simulink library "dspmtrx3"  (Simulink 6.0)
settings: Solver=ode45  SolverMode=SingleTasking  StartTime=0.0  StopTime=10.0  RelTol=1e-3
values from neighbouring files (symbols this model uses):
  a = []    [dspfdes.m]    (also in dsprprim.m = a-Mi)
undefined symbols (not defined in the file or in its folder): dTypeID
libraries: dspmtrx3 x12, simulink x3, dspsolvers x3, dspsigattribs x2, dspstat3 x1
settings Model: RequirementInfo=9  CovMetricSettings=d  Creator=szlotkin  LastModifiedBy=mlongfri  ExtModeAutoUpdateStatusClock=off  ProdHWDeviceType=Specified
settings DataIOCC: SignalLoggingName=logsOut
settings OptimizationCC: BooleanDataType=off
settings DebuggingCC: CheckExecutionContextPreStartOutputMsg=on  CheckExecutionContextRuntimeOutputMsg=on  SolverPrmCheckMsg=none
settings HardwareCC: ProdHWDeviceType=Specified  TargetUnknown=on
settings SFSimCC: SFSimApplyToAllLibs=on  SFSimBuildMode=Incremental

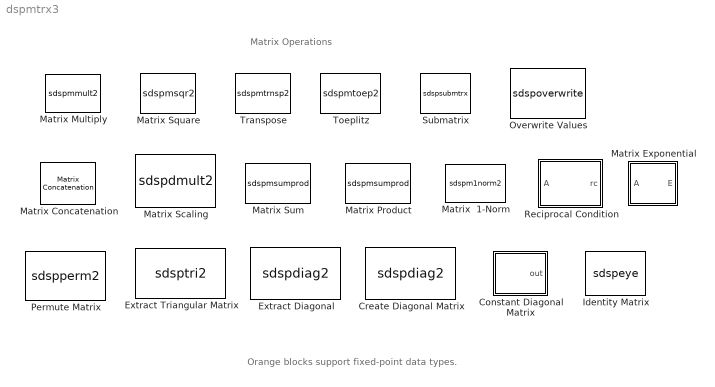
== system dspmtrx3 ==
  note: Matrix Operations
  note: Orange blocks support fixed-point data types.
  Constant Diagonal Matrix : Subsystem  PropExecContextAcrossSSBoundary=on  mask(Constant Diagonal Matrix){q=ones(1,3), frame=off, additionalParams=off, allowOverrides=on, dataType=Inherit from 'Constant(s) along diagonal', isSigned=on, wordLen=16, udDataType=sfix(16), fracBitsMode=Best precision, numFracBits=15}
      mask prompts: q "Constant(s) along diagonal:"; frame "Frame-based output"; additionalParams "------- Show additional parameters --------"; allowOverrides "Allow overrides by DSP Fixed-Point Attributes blocks"; dataType "Output data type:"; isSigned "Signed"; wordLen "Word length:"; udDataType "User-defined data type:"; fracBitsMode "Set fraction length in output to:"; numFracBits "Fraction length:"
      mask help: Generate a diagonal matrix having elements specified by a vector constant.
      mask init:
      | [a,x,y] = dspblkconstdiag('icon',q);
      | dspblkconstdiag('init');
      settings: CopyFcn=dspfixptcopycallback
      mask Help: web(dspbhelp);
      mask StyleString: edit,checkbox,checkbox,checkbox,popup(double|single|int8|uint8|int16|uint16|int32|uint32|boolean|Fixed-point|User-defined|Inherit from 'Constant(s) along diagonal'|Inherit via back propagation),checkbox,edit,edit,popup(Best precision|User-defined),edit
      mask CallbackString: ||||dspblkconstdiag;|||dspblkconstdiag;|dspblkconstdiag;|
      mask TabNameString: Main,Main,Main,Main,Data Types,Data Types,Data Types,Data Types,Data Types,Data Types
      mask Display: plot(x,y)
  Create Diagonal Matrix : S-Function  FunctionName=sdspdiag2  Parameters=mode  mask(Create Diagonal Matrix){}
      mask help: Convert a vector of diagonal elements to a full matrix.
      mask init:
      | mode = 1;
      | x = [.58 .87 .87 .58 .58 NaN 0.45 0.12 NaN 0.525 0.525 0.475 0.475 0.525 0.525 0.565 0.525 ];
      | y = [ 0.2 0.2 0.8 0.8 0.2 NaN 0.2 0.8 NaN 0.435 0.475 0.475 0.525 0.525 0.565 0.5 0.435 ];
      settings: CopyFcn=dspfixptcopycallback
      mask Help: web(dspbhelp);
      mask Display:
      | plot(x,y);
      | port_label('input',1,'D');
      | port_label('output',1,'A');
  Extract Diagonal : S-Function  FunctionName=sdspdiag2  Parameters=mode  mask(Extract Diagonal){}
      mask help: Extract the main diagonal of a full matrix.
      mask init:
      | mode = 2;
      | x = [.58 .87 NaN 0.12 0.45 0.45 0.12 0.12 NaN 0.525 0.525 0.475 0.475 0.525 0.525 0.565 0.525 ];
      | y = [ 0.8 0.2 NaN 0.2 0.2 0.8 0.8 0.2 NaN 0.435 0.475 0.475 0.525 0.525 0.565 0.5 0.435 ];
      settings: CopyFcn=dspfixptcopycallback
      mask Help: web(dspbhelp);
      mask Display:
      | plot(x,y);
      | port_label('input',1,'A');
      | port_label('output',1,'D');
  Extract Triangular Matrix : S-Function  FunctionName=sdsptri2  Parameters=fcn  mask(Extract Triangular Matrix){fcn=Upper}
      mask prompts: fcn "Extract:"
      mask help: Extract upper or lower triangular part of input matrix.
      mask init:
      | [s,x,y] = dspblktri(fcn);
      settings: CopyFcn=dspfixptcopycallback
      mask Help: web(dspbhelp);
      mask StyleString: popup(Upper|Lower)
      mask Display:
      | plot(x,y);
      | port_label('input',1,'A');
      | port_label('output',1,s);
  Identity Matrix : S-Function  FunctionName=sdspeye  Parameters=Inherit,N,Ts,isCustomFloat,isSigned,dTypeID,wordLength,fracBits,1  mask(Identity Matrix){Inherit=off, N=5, Ts=1, additionalParams=off, allowOverrides=on, dataType=double, isSigned=on, wordLen=16, udDataType=sfix(16), fracBitsMode=Best precision, numFracBits=15}
      mask prompts: Inherit "Inherit output port attributes from input port"; N "Matrix size:"; Ts "Sample time:"; additionalParams "------- Show additional parameters --------"; allowOverrides "Allow overrides by DSP Fixed-Point Attributes blocks"; dataType "Output data type:"; isSigned "Signed"; wordLen "Word length:"; udDataType "User-defined data type (e.g. sfix(16), float('single')):"; fracBitsMode "Set fraction length in output to:"; numFracBits "Fraction length:"
      mask help: Output an identity matrix. If the matrix size entered is a scalar, then the output will be a square (symmetric) identity matrix with the number of rows and columns both equal to the specified value. If the matrix size entered is a two-element vector [M N], then the output will be an asymmetric matrix with the number of rows equal to M, the number of columns equal to N, ones down the diagonal, and zeros elsewhere. This matches the syntax of the MATLAB function eye(N) and eye(M,N), respectively.
      mask init:
      | if Inherit,
      |    str = 'eye( )';
      | else
      |    str = ['eye(' ,num2str(&2),')'];
      | end
      | [dtInfo,dTypeID]=dspblkeye('init');
      | isSigned=dtInfo.DataTypeIsSigned;
      | isCustomFloat=dtInfo.DataTypeIsCustomFloat;
      | wordLength=dtInfo.DataTypeWordLength;
      | fracBits=dtInfo.DataTypeFracOrMantBits;
      settings: CopyFcn=dspfixptcopycallback
      mask Help: web(dspbhelp);
      mask StyleString: checkbox,edit,edit,checkbox,checkbox,popup(double|single|int8|uint8|int16|uint16|int32|uint32|boolean|Fixed-point|User-defined|Inherit via back propagation),checkbox,edit,edit,popup(Best precision|User-defined),edit
      mask CallbackString: dspblkeye|||||dspblkeye|||dspblkeye|dspblkeye|
      mask TabNameString: Main,Main,Main,Main,Main,Data Types,Data Types,Data Types,Data Types,Data Types,Data Types
      mask Display: disp(str)
  Matrix Concatenation : simulink/Math Operations/Matrix Concatenation  numInports=2  catMethod=Horizontal
  Matrix Exponential : Subsystem  PropExecContextAcrossSSBoundary=on
      mask Type: Matrix Exponential
      mask Description: Compute the matrix exponential, using a scaling and squaring algorithm with a Pade approximation.  Matrix must be square.
      mask Help: web(dspbhelp);
      mask Display: disp('expm')
  Matrix Product : S-Function  DialogController=dspDDGCreate  DialogControllerArgs=DataTag0  FunctionName=sdspmsumprod  Parameters=Dim,2,dtInfo.interProdMode,dtInfo.interProdWordLength,dtInfo.interProdFracLength,dtInfo.prodOutputMode,dtInfo.prodOutputWordLength,dtInfo.prodOutputFracLength,dtInfo.accumMode,dtInfo.accumWordLength,dtInfo.accumFracLength,dtInfo.outputMode,dtInfo.outputWordLength,dtInfo.outputFracLength,dtInfo.roundingMode,dtInfo.overflowMode  mask(Matrix Product){Dim=Columns, additionalParams=off, allowOverrides=on, outputMode=Same as product output, outputWordLength=16, outputFracLength=15, accumMode=Inherit via internal rule, accumWordLength=32, accumFracLength=30, prodOutputMode=Inherit via internal rule, prodOutputWordLength=32, prodOutputFracLength=30, interProdMode=Same as input, interProdWordLength=16, interProdFracLength=15, roundingMode=Floor, overflowMode=off, LockScale=off}
      mask prompts: Dim "Multiply along:"; additionalParams "------- Show additional parameters -------"; allowOverrides "Allow overrides from DSP Fixed-Point Attributes blocks"; outputMode "Fixed-point output attributes:"; outputWordLength "Output word length:"; outputFracLength "Output fraction length:"; accumMode "Fixed-point accumulator attributes:"; accumWordLength "Accumulator word length:"; accumFracLength "Accumulator fraction length:"; prodOutputMode "Fixed-point product output attributes:"; prodOutputWordLength "Product output word length:"; prodOutputFracLength "Product output fraction length:"; interProdMode "Fixed-point intermediate product attributes:"; interProdWordLength "Intermediate product word length:"; interProdFracLength "Intermediate product fraction length:"; roundingMode "Round integer calculations toward:"; overflowMode "Saturate on integer overflow"; LockScale "Lock scaling"
      mask help:
      | Product of matrix elements along the row or column dimension. Note that 1-D input signals produce a single scalar output equal to the product of the individual elements.
      |
      | The accumulator attributes are only used with complex fixed-point inputs.
      mask init:
      | if (Dim==1), str='Row\nProduct';
      | else str='Column\nProduct';
      | end
      | 
      | %misc         1 USED
      | %output       2 USED
      | %accum        4 USED
      | %prodOutput   8 USED
      | %memory      16
      | %firstCoeff  32
      | %secondCoeff 64
      | %thirdCoeff 128
      | %interProd  256 USED
      | %1+2+4+8+256 = 271
      | dtInfo = dspGetFixptDataTypeInfo(gcbh,271);
      settings: CopyFcn=dspfixptcopycallback
      mask Help: web(dspbhelp);
      mask StyleString: popup(Rows|Columns),checkbox,checkbox,popup(Same as product output|Same as input|Binary point scaling|Slope and bias scaling|User-defined),edit,edit,popup(Inherit via internal rule|Same as product output|Same as input|Binary point scaling|Slope and bias scaling|User-defined),edit,edit,popup(Inherit via internal rule|Same as input|Binary point scaling|Slope and bias scaling|User-defined),edit,edit,popup(Same as input|Binary point scaling|Slope and bias scaling|User-defined),edit,edit,popup(Floor|Nearest),checkbox,checkbox
      mask Display: disp(str);
  Matrix Scaling : S-Function  DialogController=dspDDGCreate  DialogControllerArgs=DataTag1  FunctionName=sdspdmult2  Parameters=mode,D_Source,D_VectFromMask,dtInfo.firstCoeffMode,dtInfo.firstCoeffWordLength,dtInfo.firstCoeffFracLength,dtInfo.prodOutputMode,dtInfo.prodOutputWordLength,dtInfo.prodOutputFracLength,dtInfo.accumMode,dtInfo.accumWordLength,dtInfo.accumFracLength,dtInfo.outputMode,dtInfo.outputWordLength,dtInfo.outputFracLength,dtInfo.roundingMode,dtInfo.overflowMode  mask(Matrix Scaling){mode=Scale Rows (D*A), D_Source=Input port, D_VectFromMask=[0.5 0.25], additionalParams=off, allowOverrides=on, firstCoeffMode=Same word length as input, firstCoeffWordLength=16, firstCoeffFracLength=15, outputMode=Same as product output, outputWordLength=16, outputFracLength=15, accumMode=Inherit via internal rule, accumWordLength=32, accumFracLength=30, prodOutputMode=Inherit via internal rule, prodOutputWordLength=32, prodOutputFracLength=30, roundingMode=Floor, overflowMode=off, LockScale=off}
      mask prompts: D_Source "Scaling vector (D) source:"; D_VectFromMask "Scaling vector (D):"; additionalParams "------- Show additional parameters -------"; allowOverrides "Allow overrides from DSP Fixed-Point Attributes blocks"; firstCoeffMode "Fixed-point scaling vector attributes:"; firstCoeffWordLength "Scaling vector elements word length:"; firstCoeffFracLength "Scaling vector elements fraction length:"; outputMode "Fixed-point output attributes:"; outputWordLength "Output word length:"; outputFracLength "Output fraction length:"; accumMode "Fixed-point accumulator attributes:"; accumWordLength "Accumulator word length"; accumFracLength "Accumulator fraction length:"; prodOutputMode "Fixed-point product output attributes:"; prodOutputWordLength "Product output word length:"; prodOutputFracLength "Product output fraction length:"; roundingMode "Round integer calculations toward:"; overflowMode "Saturate on integer overflow"; LockScale "Lock scaling"
      mask help:
      | Scale the columns or rows of a matrix A by the elements of a vector D.  This is equivalent to multiplying a full matrix (A) by a diagonal (D), and vice versa. Note that unoriented input signals are treated as oriented column vectors. The output of this block is always oriented.
      |
      | For some fixed-point modes, the scaling vector fraction length or slope is automatically set for you to ''Best precision.'' In these cases, the scaling is set to the best possible precision given the scaling vector real-world values and word length. This is equivalent to the ''Best Precision: Matrix-wise'' scaling option used in some Simulink fixed-point blocks.
      |
      | The accumulator attributes on the ''Fixed-point'' tab are only used with complex fixed-point inputs.
      mask init:
      | %misc         1 USED
      | %output       2 USED
      | %accum        4 USED
      | %prodOutput   8 USED
      | %memory      16
      | %firstCoeff  32 USED
      | %1+2+4+8+256 = 47
      | dtInfo = dspGetFixptDataTypeInfo(gcbh,47);
      | 
      | if (strcmp(mode,'Scale rows (D*A)'))
      |     s = 'Scale\nRows\nD*A';
      | else
      | 	s = 'Scale\nColumns\nA*D';
      | end
      | 
      | inp1_index = 1;
      | inp1_label = 'A';
      | if (D_Source == 1),
      |   inp2_index = 2;
      |   inp2_label = 'D';
      | else
      |   inp2_index = 1;
      |   inp2_label = 'A';
      | end
      settings: CopyFcn=dspfixptcopycallback
      mask Help: web(dspbhelp);
      mask StyleString: popup(Scale rows (D*A)|Scale columns (A*D)),popup(Input port|Dialog parameter),edit,checkbox,checkbox,popup(Same word length as input|Specify word length|Binary point scaling|Slope and bias scaling|User-defined),edit,edit,popup(Same as product output|Same as first input|Binary point scaling|Slope and bias scaling|User-defined),edit,edit,popup(Inherit via internal rule|Same as product output|Same as first input|Binary point scaling|Slope and bias scaling|User-defined),edit,edit,popup(Inherit via internal rule|Same as first input|Binary point scaling|Slope and bias scaling|User-defined),edit,edit,popup(Floor|Nearest),checkbox,checkbox
      mask Display:
      | port_label('input',inp1_index,inp1_label);
      | port_label('input',inp2_index,inp2_label);
      | disp(s);
  Matrix Square : S-Function  FunctionName=sdspmsqr2
      mask Type: Matrix Square
      mask Description: Compute the matrix square, U' * U.  Hermitian transpose is performed for complex inputs.  [Mx1] and [1xN] input matrices may be used to compute efficient outer and inner products, respectively. Vector input signals are treated as [Mx1] matrices. The output is always a matrix.
      mask Help: web(dspbhelp);
      mask Display: disp('u^Hu','texmode','on')
  Matrix Sum : S-Function  DialogController=dspDDGCreate  DialogControllerArgs=DataTag2  FunctionName=sdspmsumprod  Parameters=Dim,1,-1,0,0,-1,0,0,dtInfo.accumMode,dtInfo.accumWordLength,dtInfo.accumFracLength,dtInfo.outputMode,dtInfo.outputWordLength,dtInfo.outputFracLength,dtInfo.roundingMode,dtInfo.overflowMode  mask(Matrix Sum){Dim=Columns, additionalParams=off, allowOverrides=on, outputMode=Same as accumulator, outputWordLength=16, outputFracLength=15, accumMode=Inherit via internal rule, accumWordLength=32, accumFracLength=30, roundingMode=Floor, overflowMode=off, LockScale=off}
      mask prompts: Dim "Sum along:"; additionalParams "------- Show additional parameters -------"; allowOverrides "Allow overrides from DSP Fixed-Point Attributes blocks"; outputMode "Fixed-point output attributes:"; outputWordLength "Output word length:"; outputFracLength "Output fraction length:"; accumMode "Fixed-point accumulator attributes:"; accumWordLength "Accumulator word length:"; accumFracLength "Accumulator fraction length:"; roundingMode "Round integer calculations toward:"; overflowMode "Saturate on integer overflow"; LockScale "Lock scaling"
      mask help: Sum of matrix elements along the row or column dimension. Note that 1-D input signals produce a single scalar output equal to the sum of the individual elements.
      mask init:
      | if (Dim==1), str='Row\nSum';
      | else str='Column\nSum';
      | end
      | 
      | %misc       1 USED
      | %output     2 USED
      | %accum      4 USED
      | dtInfo = dspGetFixptDataTypeInfo(gcbh,7);
      settings: CopyFcn=dspfixptcopycallback
      mask Help: web(dspbhelp);
      mask StyleString: popup(Rows|Columns),checkbox,checkbox,popup(Same as accumulator|Same as input|Binary point scaling|Slope and bias scaling|User-defined),edit,edit,popup(Inherit via internal rule|Same as input|Binary point scaling|Slope and bias scaling|User-defined),edit,edit,popup(Floor|Nearest),checkbox,checkbox
      mask Display: disp(str);
  Matrix  1-Norm : S-Function  DialogController=dspDDGCreate  DialogControllerArgs=DataTag3  FunctionName=sdspm1norm2  Parameters=dtInfo.accumMode,dtInfo.accumWordLength,dtInfo.accumFracLength,dtInfo.outputMode,dtInfo.outputWordLength,dtInfo.outputFracLength,dtInfo.roundingMode,dtInfo.overflowMode  mask(Matrix 1-Norm){allowOverrides=on, outputMode=Same as accumulator, outputWordLength=16, outputFracLength=15, accumMode=Inherit via internal rule, accumWordLength=32, accumFracLength=30, roundingMode=Floor, overflowMode=off, LockScale=off}
      mask prompts: allowOverrides "Allow overrides from DSP Fixed-Point Attributes blocks"; outputMode "Fixed-point output attributes:"; outputWordLength "Output word length:"; outputFracLength "Output fraction length:"; accumMode "Fixed-point accumulator attributes:"; accumWordLength "Accumulator word length:"; accumFracLength "Accumulator fraction length:"; roundingMode "Round integer calculations toward:"; overflowMode "Saturate on integer overflow"; LockScale "Lock scaling"
      mask help: Compute the matrix 1-norm, which is the largest column sum of absolute values. Note that unoriented input signals are treated as oriented column vectors. The output of this block is always oriented.
      mask init:
      | dtInfo = dspGetFixptDataTypeInfo(gcbh,7);
      settings: CopyFcn=dspfixptcopycallback
      mask Help: web(dspbhelp);
      mask StyleString: checkbox,popup(Same as accumulator|Same as input|Binary point scaling|Slope and bias scaling|User-defined),edit,edit,popup(Inherit via internal rule|Same as input|Binary point scaling|Slope and bias scaling|User-defined),edit,edit,popup(Floor|Nearest),checkbox,checkbox
      mask Display: disp('Matrix\n1-Norm')
  Matrix Multiply : S-Function  FunctionName=sdspmmult2  Parameters=numInputPorts,OptimizationLevel  mask(Matrix Multiply){numInputPorts=2, OptimizationLevel=None}
      mask prompts: numInputPorts "Number of input ports:"; OptimizationLevel "Optimization:"
      mask help: Multiply input matrices.
      mask init:
      | dspblkmmult(numInputPorts);
      mask Help: web(dspbhelp);
      mask StyleString: edit,popup(None|Memory|Flops)
      mask Display: port_label('input',1, 'A'); port_label('input',2, 'B'); port_label('output', 1, 'A*B');
  Overwrite Values : S-Function  FunctionName=sdspoverwrite  Parameters=ColSpan, ColStartMode, ColStartIndex, ColEndMode, ColEndIndex, RowSpan, RowStartMode, RowStartIndex, RowEndMode, RowEndIndex, OverWriteDiag, ConstValue, DiagSpan, DiagStartMode, DiagStartIndex, DiagEndMode, DiagEndIndex, valFrom2ndIP  mask(Overwrite Values){OverWriteDiag=Submatrix, valFrom2ndIP=Specify via dialog, ConstValue=0, RowSpan=Range of rows, RowStartMode=First, RowStartIndex=1, RowEndMode=Last, RowEndIndex=1, ColSpan=Range of columns, ColStartMode=First, ColStartIndex=1, ColEndMode=Last, ColEndIndex=1, DiagSpan=Range of elements, DiagStartMode=Index, DiagStartIndex=2, DiagEndMode=Index, DiagEndIndex=4}
      mask prompts: OverWriteDiag "Overwrite:"; valFrom2ndIP "Source of overwriting value(s):"; ConstValue "Overwrite with:"; RowSpan "Row span:"; RowStartMode "Starting row:"; RowStartIndex "Starting row index:"; RowEndMode "Ending row:"; RowEndIndex "Ending row index:"; ColSpan "Column span:"; ColStartMode "Starting column:"; ColStartIndex "Starting column index:"; ColEndMode "Ending column:"; ColEndIndex "Ending column index:"; DiagSpan "Diagonal span:"; DiagStartMode "Starting element:"; DiagStartIndex "Starting element index:"; DiagEndMode "Ending element:"; DiagEndIndex "Ending element index:"
      mask help:
      | Overwrites a selected portion of the input matrix--either a submatrix, full diagonal, or a portion of the diagonal.
      | Specify overwriting values as follows:
      |   --Matrix with the same dimensions as the submatrix
      |   --Vector with the same length as the portion of the diagonal
      |   --Scalar constant with which to replace each element in the submatrix or diagonal portion.
      |
      | Treats unoriented (1-D) input vectors as column vectors.
      mask init:
      | [x1,y1,xc,yc,xmc,ymc,xi,yi] = dspblkoverwrite('icon');
      | if valFrom2ndIP == 1
      |   i1=1;
      |   s1='';
      | else
      |   i1=2;
      |   s1='V';
      | end;
      settings: CopyFcn=dspfixptcopycallback
      mask Help: web(dspbhelp);
      mask StyleString: popup(Submatrix|Diagonal),popup(Specify via dialog|Second input port),edit,popup(All rows|One row|Range of rows),popup(First|Index|Offset from last|Last|Offset from middle|Middle),edit,popup(Index|Offset from last|Last|Offset from middle|Middle),edit,popup(All columns|One column|Range of columns),popup(First|Index|Offset from last|Last|Offset from middle|Middle),edit,popup(Index|Offset from last|Last|Offset from middle|Middle),edit,popup(All elements|One element|Range of elements),popup(First|Index|Offset from last|Last|Offset from middle|Middle),edit,popup(Index|Offset from last|Last|Offset from middle|Middle),edit
      mask CallbackString:
      | dspblkoverwrite;
      | dspblkoverwrite('icon');|dspblkoverwrite||dspblkoverwrite|dspblkoverwrite||dspblkoverwrite||dspblkoverwrite|dspblkoverwrite||dspblkoverwrite||dspblkoverwrite|dspblkoverwrite||dspblkoverwrite|
      mask Display:
      | plot(x1,y1,xc,yc,xmc,ymc,xi,yi);
      | port_label('input',1,'A');
      | port_label('output',1,'B');
      | port_label('input',i1,s1);
  Permute Matrix : S-Function  FunctionName=sdspperm2  Parameters=mode,errmode,checkDims, ZeroOneIdxMode  mask(Permute Matrix){mode=Columns, ZeroOneIdxMode=One-based, errmode=Clip Index, checkDims=off}
      mask prompts: mode "Permute:"; ZeroOneIdxMode "Index mode:"; errmode "Invalid permutation index:"; checkDims "Error when length of P is not equal to Permute dimension size"
      mask help: Permutes the rows or columns of a matrix or vector A, based on a vector P of integer-valued permutation indices. The indices need not be unique. When you select the Error check box, the length of vector P must be the same as the number of input rows or columns (whichever you are permuting).
      settings: CopyFcn=dspfixptcopycallback
      mask Help: web(dspbhelp);
      mask StyleString: popup(Rows|Columns),popup(Zero-based|One-based),popup(Clip Index|Clip and Warn|Generate Error),checkbox
      mask Display:
      | disp(['Permute\n' &1]);
      | port_label('input',1,'A');
      | port_label('input',2,'P');
  Reciprocal Condition : Subsystem  PropExecContextAcrossSSBoundary=on
      mask Type: Reciprocal Condition
      mask Description: Estimates the reciprocal of the condition of a square input matrix in the 1-norm.  If input is well conditioned, the output is near 1.0.  If input is badly conditioned, output is near 0.0.
      mask Help: web(dspbhelp);
      mask Display: disp('RCond')
  Submatrix : S-Function  FunctionName=sdspsubmtrx  Parameters=ColSpan, ColStartMode, ColStartIndex, ColEndMode, ColEndIndex, RowSpan, RowStartMode, RowStartIndex, RowEndMode, RowEndIndex  mask(Submatrix){RowSpan=Range of rows, RowStartMode=First, RowStartIndex=1, RowEndMode=Last, RowEndIndex=1, ColSpan=Range of columns, ColStartMode=First, ColStartIndex=1, ColEndMode=Last, ColEndIndex=1}
      mask prompts: RowSpan "Row span:"; RowStartMode "Starting row:"; RowStartIndex "Starting row index:"; RowEndMode "Ending row:"; RowEndIndex "Ending row index:"; ColSpan "Column span:"; ColStartMode "Starting column:"; ColStartIndex "Starting column index:"; ColEndMode "Ending column:"; ColEndIndex "Ending column index:"
      mask help: Return selected portion of input matrix. 1-D input signals are treated as 2-D column vectors. The output is always 2-D.
      mask init:
      | [x1,y1,xc,yc,xi,yi] = dspblksubmatrix('icon');
      settings: CopyFcn=dspfixptcopycallback
      mask Help: web(dspbhelp);
      mask StyleString: popup(All rows|One row|Range of rows),popup(First|Index|Offset from last|Last|Offset from middle|Middle),edit,popup(Index|Offset from last|Last|Offset from middle|Middle),edit,popup(All columns|One column|Range of columns),popup(First|Index|Offset from last|Last|Offset from middle|Middle),edit,popup(Index|Offset from last|Last|Offset from middle|Middle),edit
      mask CallbackString: dspblksubmatrix|dspblksubmatrix||dspblksubmatrix||dspblksubmatrix|dspblksubmatrix||dspblksubmatrix|
      mask Display: plot(x1,y1,xc,yc,xi,yi);
  Toeplitz : S-Function  FunctionName=sdspmtoep2  Parameters=Symmetric,1,overflowFlag+1  mask(Toeplitz){Symmetric=on, overflowFlag=on}
      mask prompts: overflowFlag "Saturate on integer overflow"
      mask help: Generate a symmetric or asymmetric Toeplitz matrix. If Symmetric is selected, a symmetric (or Hermitian) Toeplitz matrix is generated. If Symmetric is not selected, an asymmetric Toeplitz matrix is generated. The columns and rows are specified by the first and second inputs, respectively. The first matrix element is inherited from the column.
      mask init:
      | if (Symmetric==1)
      |   % Do not display anything on ports for this case
      |   p1 = 1; L1 = '';
      |   p2 = 1;  L2 = '';
      |   % Icon display is diagonal matrix picture
      |   horiz_offset = 0.1;
      |   xm=horiz_offset + .8*[0.25 0.1625 0.1625 0.25 NaN 0.7875 0.8875 0.8875 0.7875 NaN 0.25 0.75 NaN 0.4125 0.75 NaN 0.5875 0.75 NaN 0.25 0.5875 NaN 0.25 0.4125];
      |   ym=[.9 .9 .1 .1 NaN .9 .9 .1 .1 NaN .8 .2 NaN .8 .4 NaN .8 .6 NaN .6 .2 NaN .4 .2];
      | else
      |   p1 = 1;  L1 = 'Toep Col';
      |   p2 = 2;  L2 = 'Toep Row';
      |   % Icon display is blank
      |   xm = 0;
      |   ym = 0;
      | end
      settings: CopyFcn=dspfixptcopycallback
      mask Help: web(dspbhelp);
      mask CallbackString:
      | if (strcmp(get_param(gcbh,'Symmetric'),'on'))
      | 	set_param(gcbh,'MaskVisibilities',{'on','on'})
      | else
      | 	set_param(gcbh,'MaskVisibilities',{'on','off'})
      | end|
      mask Display:
      | plot(xm,ym);
      | port_label('input', p1, L1);
      | port_label('input', p2, L2);
  Transpose : S-Function  FunctionName=sdspmtrnsp2  Parameters=Hermitian,1,overflowFlag+1  mask(Transpose){Hermitian=off, overflowFlag=on}
      mask prompts: overflowFlag "Saturate on integer overflow"
      mask help: Compute the matrix transpose. Vector input signals are treated as [Mx1] matrices. The output is always a matrix.
      mask init:
      | if(Hermitian==1),  str = 'u^H';
      | else               str = 'u^T';
      | end
      settings: CopyFcn=dspfixptcopycallback
      mask Help: web(dspbhelp);
      mask CallbackString:
      | if (strcmp(get_param(gcbh,'Hermitian'),'on'))
      | 	set_param(gcbh,'MaskVisibilities',{'on','on'});
      | else
      | 	set_param(gcbh,'MaskVisibilities',{'on','off'});
      | end|
      mask Display: disp(str,'texmode','on')

== system dspmtrx3/Constant Diagonal Matrix ==
  Constant : Constant  Value=a
  Frame Status Conversion : dspsigattribs/Frame Status Conversion  growRefPort=off  outframe=Sample-based
  out : Outport  InitialOutput=0
  wires:
  Constant/1 -> Frame Status Conversion/1
  Frame Status Conversion/1 -> out/1

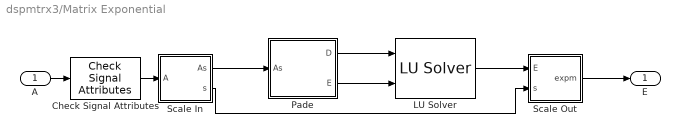
== system dspmtrx3/Matrix Exponential ==
  A : Inport  LatchInput=off
  Check Signal Attributes : dspsigattribs/Check Signal Attributes  SigAttribCheckMethod=Does not match attributes exactly  Complexity=Ignore  Frame=Sample-based  DimsCheckMethod=Is...  Dimensions=Square matrix (2-D)  DatatypeCheckMethod=Is...  DatatypeGeneral=Floating-point  DtypeFloatSpecific=Any floating-point  DtypeFixedSpecific=Any fixed-point  DtypeIntSpecific=Any integer  SampleMode=Ignore
  LU Solver : dspsolvers/LU Solver
  Pade : Subsystem  PropExecContextAcrossSSBoundary=on
      mask Display: disp('Pade\nApprox')
  Scale In : Subsystem  PropExecContextAcrossSSBoundary=on
  Scale Out : Subsystem  PropExecContextAcrossSSBoundary=on
  E : Outport
  wires:
  Check Signal Attributes/1 -> Scale In/1(A)
  A/1 -> Check Signal Attributes/1
  Scale In/1(As) -> Pade/1(As)
  Scale Out/1(expm) -> E/1
  Scale In/2(s) -> Scale Out/2(s)
  Pade/2(E) -> LU Solver/2
  Pade/1(D) -> LU Solver/1
  LU Solver/1 -> Scale Out/1(E)

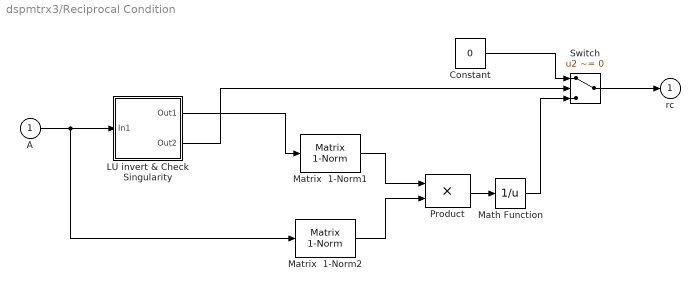
== system dspmtrx3/Reciprocal Condition ==
  A : Inport  LatchInput=off
  Constant : Constant  Value=0
  LU invert & Check Singularity : Subsystem  PropExecContextAcrossSSBoundary=on
      mask Display:
      | port_label('output',1,'Inv');
      | port_label('output',2,'Status');
      | port_label('input',1,'Mx');
  Math Function : Math  Operator=reciprocal  SaturateOnIntegerOverflow=on
  Matrix  1-Norm1 : dspmtrx3/Matrix  1-Norm
  Matrix  1-Norm2 : dspmtrx3/Matrix  1-Norm
  Product : Product  SaturateOnIntegerOverflow=on  InputSameDT=on
  Switch : Switch  Criteria=u2 ~= 0  InputSameDT=on
  " rc" : Outport  InitialOutput=0
  wires:
  LU invert & Check Singularity/2(Out2) -> Switch/2
  Math Function/1 -> Switch/3
  Switch/1 -> " rc"/1
  Product/1 -> Math Function/1
  Matrix  1-Norm2/1 -> Product/2
  Matrix  1-Norm1/1 -> Product/1
  Constant/1 -> Switch/1
  LU invert & Check Singularity/1(Out1) -> Matrix  1-Norm1/1
  A/1 -> LU invert & Check Singularity/1(In1), Matrix  1-Norm2/1

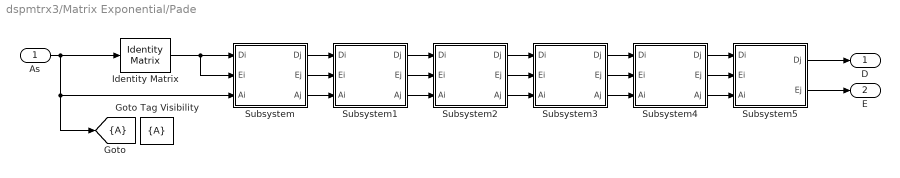
== system dspmtrx3/Matrix Exponential/Pade ==
  As : Inport  LatchInput=off
  Goto Tag Visibility : GotoTagVisibility
  Identity Matrix : dspmtrx3/Identity Matrix  Inherit=on  N=5  Ts=1  dataType=double  wordLen=16  udDataType=sfix(16)  fracBitsMode=Best precision  numFracBits=15
  Subsystem : Subsystem  PropExecContextAcrossSSBoundary=on
      mask Display: disp('Pade\n1')
  Subsystem1 : Subsystem  PropExecContextAcrossSSBoundary=on
      mask Display: disp('Pade\n2')
  Subsystem2 : Subsystem  PropExecContextAcrossSSBoundary=on
      mask Display: disp('Pade\n3')
  Subsystem3 : Subsystem  PropExecContextAcrossSSBoundary=on
      mask Display: disp('Pade\n4')
  Subsystem4 : Subsystem  PropExecContextAcrossSSBoundary=on
      mask Display: disp('Pade\n5')
  Subsystem5 : Subsystem  PropExecContextAcrossSSBoundary=on
      mask Display: disp('Pade\n6')
  D : Outport
  E : Outport  Port=2
  tag scope: A=scoped
  wires:
  As/1 -> Identity Matrix/1, Subsystem/3(Ai), [A]
  Identity Matrix/1 -> Subsystem/1(Di), Subsystem/2(Ei)
  Subsystem/1(Dj) -> Subsystem1/1(Di)
  Subsystem/2(Ej) -> Subsystem1/2(Ei)
  Subsystem1/1(Dj) -> Subsystem2/1(Di)
  Subsystem1/2(Ej) -> Subsystem2/2(Ei)
  Subsystem2/1(Dj) -> Subsystem3/1(Di)
  Subsystem2/2(Ej) -> Subsystem3/2(Ei)
  Subsystem3/1(Dj) -> Subsystem4/1(Di)
  Subsystem3/2(Ej) -> Subsystem4/2(Ei)
  Subsystem4/1(Dj) -> Subsystem5/1(Di)
  Subsystem4/2(Ej) -> Subsystem5/2(Ei)
  Subsystem5/2(Ej) -> E/1
  Subsystem5/1(Dj) -> D/1
  Subsystem/3(Aj) -> Subsystem1/3(Ai)
  Subsystem1/3(Aj) -> Subsystem2/3(Ai)
  Subsystem2/3(Aj) -> Subsystem3/3(Ai)
  Subsystem3/3(Aj) -> Subsystem4/3(Ai)
  Subsystem4/3(Aj) -> Subsystem5/3(Ai)

== system dspmtrx3/Matrix Exponential/Scale In ==
  A : Inport  LatchInput=off
  Inf norm : Subsystem  PropExecContextAcrossSSBoundary=on
      mask Display: disp('inf\nnorm')
  Pow2 Scaling : Subsystem  PropExecContextAcrossSSBoundary=on
      mask Display: disp('s-scaling')
  Scale Input : Subsystem  PropExecContextAcrossSSBoundary=on
  log2 : Subsystem  PropExecContextAcrossSSBoundary=on
      mask Display: disp('log2')
  As : Outport
  s : Outport  Port=2
  wires:
  A/1 -> Inf norm/1(In1), Scale Input/2(A)
  Inf norm/1(Out1) -> log2/1(u)
  log2/1(e) -> Pow2 Scaling/1(In1)
  Pow2 Scaling/1(Out1) -> Scale Input/1(s), s/1
  Scale Input/1(sA) -> As/1

== system dspmtrx3/Matrix Exponential/Scale Out ==
  E : Inport  LatchInput=off
  s : Inport  Port=2  LatchInput=off
  Matrix Squaring : Subsystem  TreatAsAtomicUnit=on  PropExecContextAcrossSSBoundary=on
  Switch : Switch  Criteria=u2 ~= 0  SaturateOnIntegerOverflow=on
  expm : Outport
  wires:
  s/1 -> Matrix Squaring/2(N), Switch/2
  E/1 -> Matrix Squaring/1(E), Switch/3
  Matrix Squaring/1(Out) -> Switch/1
  Switch/1 -> expm/1

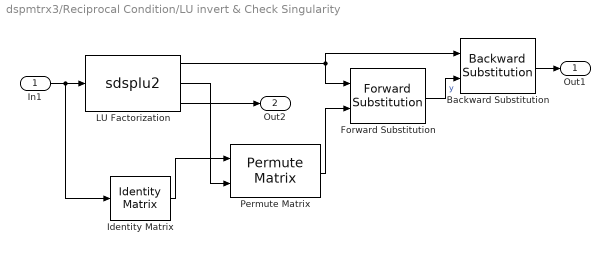
== system dspmtrx3/Reciprocal Condition/LU invert & Check Singularity ==
  In1 : Inport  LatchInput=off
  Backward Substitution : dspsolvers/Backward Substitution  unit=off
  Forward Substitution : dspsolvers/Forward Substitution  unit=on
  Identity Matrix : dspmtrx3/Identity Matrix  Inherit=on  N=5  Ts=1  dataType=double  wordLen=16  udDataType=sfix(16)  fracBitsMode=Best precision  numFracBits=15
  LU Factorization : S-Function  AncestorBlock=dspfactors/LU Factorization  FunctionName=sdsplu2  Parameters=singular  mask(LU Factorization){singular=on}
      mask prompts: singular "Show singularity  status"
      mask help: LU factorization with row pivoting. Only for use with a square input matrix A. Stores L (a unit-lower triangular matrix) in the lower triangle and U in the upper triangle of the output matrix. Permutation vector P is output separately.
      mask init:
      | x=[ 0.58 0.85 0.58 0.58 NaN 0.895 0.625 0.895 0.895 NaN 0.12 0.45 0.45 0.12 0.12 NaN 0.525 0.525 0.475 0.475 0.525 0.525 0.565 0.525 ];
      | y=[ 0.1 0.1 0.7 0.1 NaN 0.1 0.7 0.7 0.1 NaN 0.1 0.1 0.7 0.7 0.1 NaN 0.335 0.375 0.375 0.425 0.425 0.465 0.4 0.335 ];
      mask Help: web(dspbhelp);
      mask Display:
      | plot(x,y); text(.25,0.9,'P A = L U')
      | port_label('input',1,'A');
      | port_label('output',1,'LU');
      | port_label('output',2,'P');
      | port_label('output',3,'S');
  Permute Matrix : dspmtrx3/Permute Matrix  mode=Rows  ZeroOneIdxMode=One-based  errmode=Clip Index  checkDims=on
  Out1 : Outport
  Out2 : Outport  Port=2
  wires:
  LU Factorization/3 -> Out2/1
  LU Factorization/2 -> Permute Matrix/2
  LU Factorization/1 -> Backward Substitution/1, Forward Substitution/1
  Backward Substitution/1 -> Out1/1
  In1/1 -> LU Factorization/1, Identity Matrix/1
  Forward Substitution/1 -> Backward Substitution/2  "y"
  Permute Matrix/1 -> Forward Substitution/2
  Identity Matrix/1 -> Permute Matrix/1

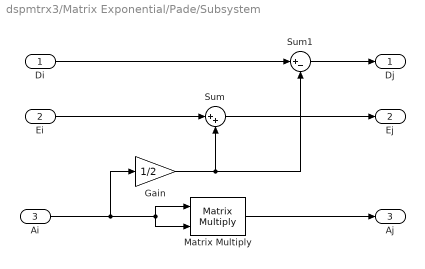
== system dspmtrx3/Matrix Exponential/Pade/Subsystem ==
  Di : Inport  LatchInput=off
  Ei : Inport  Port=2  LatchInput=off
  Ai : Inport  Port=3  LatchInput=off
  Gain : Gain  Gain=1/2  ParameterDataType=float('single')  SaturateOnIntegerOverflow=on
  Matrix Multiply : dspmtrx3/Matrix Multiply  numInputPorts=2  OptimizationLevel=None
  Sum : Sum  Inputs=|++  SaturateOnIntegerOverflow=on
  Sum1 : Sum  Inputs=|+-  SaturateOnIntegerOverflow=on
  Dj : Outport
  Ej : Outport  Port=2
  Aj : Outport  Port=3
  wires:
  Ei/1 -> Sum/1
  Sum/1 -> Ej/1
  Sum1/1 -> Dj/1
  Di/1 -> Sum1/1
  Gain/1 -> Sum/2, Sum1/2
  Ai/1 -> Gain/1, Matrix Multiply/2, Matrix Multiply/1
  Matrix Multiply/1 -> Aj/1

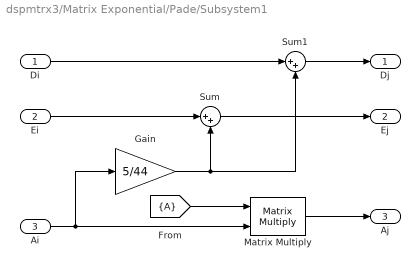
== system dspmtrx3/Matrix Exponential/Pade/Subsystem1 ==
  Di : Inport  LatchInput=off
  Ei : Inport  Port=2  LatchInput=off
  Ai : Inport  Port=3  LatchInput=off
  Gain : Gain  Gain=5/44
  Matrix Multiply : dspmtrx3/Matrix Multiply  numInputPorts=2  OptimizationLevel=None
  Sum : Sum  Inputs=|++  SaturateOnIntegerOverflow=on
  Sum1 : Sum  Inputs=|++  SaturateOnIntegerOverflow=on
  Dj : Outport
  Ej : Outport  Port=2
  Aj : Outport  Port=3
  wires:
  Di/1 -> Sum1/1
  Sum1/1 -> Dj/1
  Sum/1 -> Ej/1
  Ei/1 -> Sum/1
  Gain/1 -> Sum/2, Sum1/2
  Ai/1 -> Gain/1, Matrix Multiply/2
  Matrix Multiply/1 -> Aj/1
  [A] -> Matrix Multiply/1

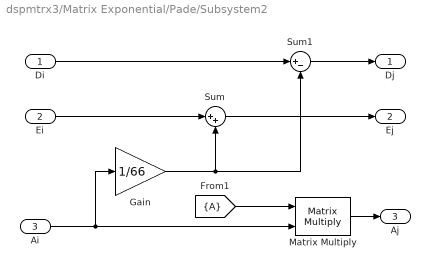
== system dspmtrx3/Matrix Exponential/Pade/Subsystem2 ==
  Di : Inport  LatchInput=off
  Ei : Inport  Port=2  LatchInput=off
  Ai : Inport  Port=3  LatchInput=off
  Gain : Gain  Gain=1/66
  Matrix Multiply : dspmtrx3/Matrix Multiply  numInputPorts=2  OptimizationLevel=None
  Sum : Sum  Inputs=|++  SaturateOnIntegerOverflow=on
  Sum1 : Sum  Inputs=|+-  SaturateOnIntegerOverflow=on
  Dj : Outport
  Ej : Outport  Port=2
  Aj : Outport  Port=3
  wires:
  Gain/1 -> Sum1/2, Sum/2
  Di/1 -> Sum1/1
  Sum1/1 -> Dj/1
  Sum/1 -> Ej/1
  Ei/1 -> Sum/1
  Ai/1 -> Matrix Multiply/2, Gain/1
  [A] -> Matrix Multiply/1
  Matrix Multiply/1 -> Aj/1

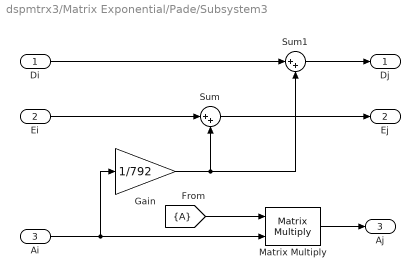
== system dspmtrx3/Matrix Exponential/Pade/Subsystem3 ==
  Di : Inport  LatchInput=off
  Ei : Inport  Port=2  LatchInput=off
  Ai : Inport  Port=3  LatchInput=off
  Gain : Gain  Gain=1/792
  Matrix Multiply : dspmtrx3/Matrix Multiply  numInputPorts=2  OptimizationLevel=None
  Sum : Sum  Inputs=|++  SaturateOnIntegerOverflow=on
  Sum1 : Sum  Inputs=|++  SaturateOnIntegerOverflow=on
  Dj : Outport
  Ej : Outport  Port=2
  Aj : Outport  Port=3
  wires:
  Gain/1 -> Sum1/2, Sum/2
  Ei/1 -> Sum/1
  Sum/1 -> Ej/1
  Sum1/1 -> Dj/1
  Di/1 -> Sum1/1
  Ai/1 -> Matrix Multiply/2, Gain/1
  Matrix Multiply/1 -> Aj/1
  [A] -> Matrix Multiply/1

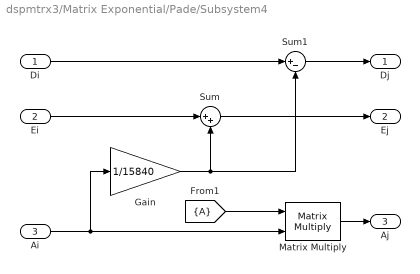
== system dspmtrx3/Matrix Exponential/Pade/Subsystem4 ==
  Di : Inport  LatchInput=off
  Ei : Inport  Port=2  LatchInput=off
  Ai : Inport  Port=3  LatchInput=off
  Gain : Gain  Gain=1/15840
  Matrix Multiply : dspmtrx3/Matrix Multiply  numInputPorts=2  OptimizationLevel=None
  Sum : Sum  Inputs=|++  SaturateOnIntegerOverflow=on
  Sum1 : Sum  Inputs=|+-  SaturateOnIntegerOverflow=on
  Dj : Outport
  Ej : Outport  Port=2
  Aj : Outport  Port=3
  wires:
  Ei/1 -> Sum/1
  Sum/1 -> Ej/1
  Sum1/1 -> Dj/1
  Di/1 -> Sum1/1
  Gain/1 -> Sum/2, Sum1/2
  Ai/1 -> Matrix Multiply/2, Gain/1
  [A] -> Matrix Multiply/1
  Matrix Multiply/1 -> Aj/1

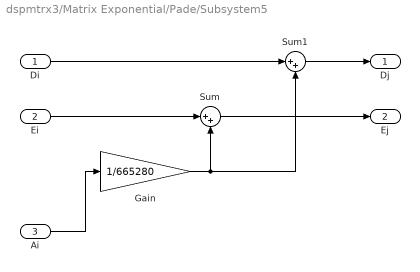
== system dspmtrx3/Matrix Exponential/Pade/Subsystem5 ==
  Di : Inport  LatchInput=off
  Ei : Inport  Port=2  LatchInput=off
  Ai : Inport  Port=3  LatchInput=off
  Gain : Gain  Gain=1/665280
  Sum : Sum  Inputs=|++  SaturateOnIntegerOverflow=on
  Sum1 : Sum  Inputs=|++  SaturateOnIntegerOverflow=on
  Dj : Outport
  Ej : Outport  Port=2
  wires:
  Di/1 -> Sum1/1
  Sum1/1 -> Dj/1
  Sum/1 -> Ej/1
  Ei/1 -> Sum/1
  Gain/1 -> Sum/2, Sum1/2
  Ai/1 -> Gain/1

== system dspmtrx3/Matrix Exponential/Scale In/Inf norm ==
  In1 : Inport  LatchInput=off
  Abs : Abs  SaturateOnIntegerOverflow=on
  Math Function : Math  Operator=conj  SaturateOnIntegerOverflow=on
  Matrix Sum : dspmtrx3/Matrix Sum  Dim=Rows  roundingMode=Floor  overflowMode=off
  Maximum : dspstat3/Maximum  fcn=Value  reset=None  roundingMode=Floor  overflowMode=off
  Out1 : Outport
  wires:
  Matrix Sum/1 -> Abs/1
  In1/1 -> Math Function/1
  Maximum/1 -> Out1/1
  Math Function/1 -> Matrix Sum/1
  Abs/1 -> Maximum/1

== system dspmtrx3/Matrix Exponential/Scale In/Pow2 Scaling ==
  In1 : Inport  LatchInput=off
  Constant : Constant  Value=0  VectorParams1D=off  OutDataTypeMode=int32
  Constant1 : Constant  VectorParams1D=off  OutDataTypeMode=int32
  MinMax : MinMax  Function=max  Inputs=2  SaturateOnIntegerOverflow=on  InputSameDT=on
  Sum : Sum  Inputs=++|  SaturateOnIntegerOverflow=on
  Out1 : Outport
  wires:
  Sum/1 -> MinMax/1
  Constant/1 -> MinMax/2
  In1/1 -> Sum/2
  MinMax/1 -> Out1/1
  Constant1/1 -> Sum/1

== system dspmtrx3/Matrix Exponential/Scale In/Scale Input ==
  s : Inport  LatchInput=off
  A : Inport  Port=2  LatchInput=off
  Data Type Conversion : DataTypeConversion  SaturateOnIntegerOverflow=on  RndMeth=Zero
  Math Function : Math  Operator=reciprocal  SaturateOnIntegerOverflow=on
  Product : Product  SaturateOnIntegerOverflow=on
  Two^N : Subsystem  PropExecContextAcrossSSBoundary=on
      mask Display: disp('2.^N')
  sA : Outport
  wires:
  Two^N/1(Out) -> Data Type Conversion/1
  Data Type Conversion/1 -> Math Function/1
  s/1 -> Two^N/1(N)
  Product/1 -> sA/1
  Math Function/1 -> Product/2
  A/1 -> Product/1

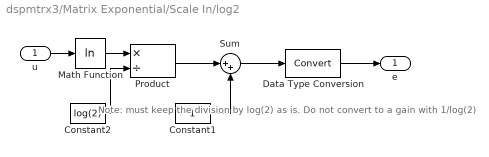
== system dspmtrx3/Matrix Exponential/Scale In/log2 ==
  note: Note: must keep the division
      | by log(2) as is.  Do not convert
      | to a gain with 1/log(2)
  u : Inport  LatchInput=off
  Constant1 : Constant  VectorParams1D=off
  Constant2 : Constant  Value=log(2)  VectorParams1D=off
  Data Type Conversion : DataTypeConversion  OutDataTypeMode=int32  SaturateOnIntegerOverflow=on  RndMeth=Zero
  Math Function : Math  Operator=log  SaturateOnIntegerOverflow=on
  Product : Product  Inputs=*/  SaturateOnIntegerOverflow=on
  Sum : Sum  Inputs=|++  RndMeth=Ceiling
  e : Outport
  wires:
  Constant2/1 -> Product/2
  Math Function/1 -> Product/1
  u/1 -> Math Function/1
  Data Type Conversion/1 -> e/1
  Product/1 -> Sum/1
  Sum/1 -> Data Type Conversion/1
  Constant1/1 -> Sum/2

== system dspmtrx3/Matrix Exponential/Scale Out/Matrix Squaring ==
  E : Inport  LatchInput=off
  N : Inport  Port=2  LatchInput=off
  For Iterator : ForIterator  ResetStates=reset  IterationSource=external
  Matrix Multiply : dspmtrx3/Matrix Multiply  numInputPorts=2  OptimizationLevel=None
  Switch : Switch  Criteria=u2 > Threshold  Threshold=1  SaturateOnIntegerOverflow=on
  Unit Delay : UnitDelay  Orientation=left  SampleTime=-1
  Out : Outport
  wires:
  N/1 -> For Iterator/1
  E/1 -> Switch/3
  For Iterator/1 -> Switch/2
  Unit Delay/1 -> Switch/1
  Matrix Multiply/1 -> Unit Delay/1, Out/1
  Switch/1 -> Matrix Multiply/1, Matrix Multiply/2

== system dspmtrx3/Matrix Exponential/Scale In/Scale Input/Two^N ==
  note: Compensate
      | for 1-based loops
  N : Inport  LatchInput=off
  2^N : Subsystem  TreatAsAtomicUnit=on  PropExecContextAcrossSSBoundary=on
  Constant : Constant  VectorParams1D=off
  Sum : Sum  Inputs=|++  SaturateOnIntegerOverflow=on
  Out : Outport
  wires:
  Constant/1 -> Sum/2
  Sum/1 -> 2^N/1(N)
  N/1 -> Sum/1
  2^N/1(Out) -> Out/1

== system dspmtrx3/Matrix Exponential/Scale In/Scale Input/Two^N/2^N ==
  N : Inport  LatchInput=off
  Bitwise Logical Operator2 : simulink/Math Operations/Bitwise Logical Operator  Operator=SHIFT_LEFT  Operand2=1
  For Iterator : ForIterator  ResetStates=reset  IterationSource=external  ShowIterationPort=off
  Signal Specification : simulink/Signal Attributes/Signal Specification  D=-1  Ts=-1  DataType=uint32  OutDataType=sfix(16)  OutScaling=2^0
      settings: SignalType=auto  SamplingMode=auto
  Unit Delay : UnitDelay  X0=uint32(1)  SampleTime=-1
  Out : Outport
  wires:
  N/1 -> For Iterator/1
  Unit Delay/1 -> Out/1, Signal Specification/1
  Bitwise Logical Operator2/1 -> Unit Delay/1
  Signal Specification/1 -> Bitwise Logical Operator2/1
